simulink model "fsm_observer"  (R2025b)
settings: Solver=ode4  StartTime=0.0  StopTime=fsm_Tstop  FixedStep=fsm_h  RelTol=1e-3
values from neighbouring files (symbols this model uses):
  fsm_L1 = 0.25 * wind_p.C'    [build_fsm_observer.m]
  fsm_L2 = 0.25 * wind_p.C'    [build_fsm_observer.m]
  fsm_S = 0.05 * wind_p.C'    [build_fsm_observer.m]
  fsm_xhat0 = zeros(6, 1)    [build_fsm_observer.m]
  wind_p = wind_plant_parameters()    [build_fsm_observer.m]
settings Model: Creator=yuexi  LastModifiedBy=yuexi

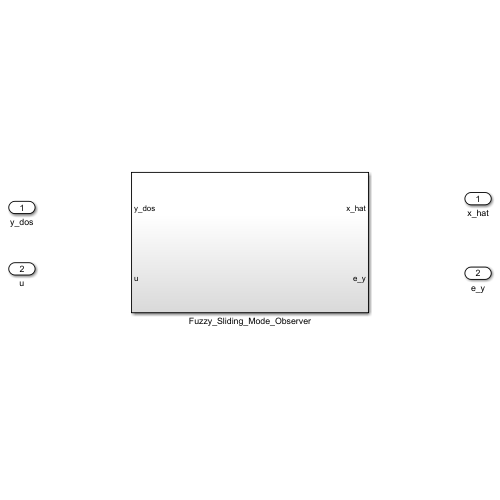
[thumbnail: Simulink's stored preview of the top-level diagram]
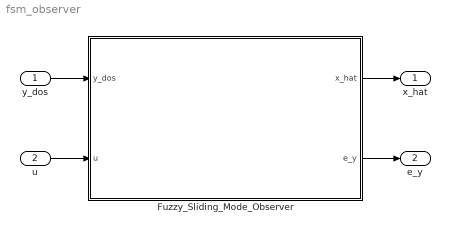
== system fsm_observer ==
  y_dos : Inport
  u : Inport  Port=2
  Fuzzy_Sliding_Mode_Observer : Subsystem
  x_hat : Outport
  e_y : Outport  Port=2
  wires:
  u/1 -> Fuzzy_Sliding_Mode_Observer/2(u)
  y_dos/1 -> Fuzzy_Sliding_Mode_Observer/1(y_dos)
  Fuzzy_Sliding_Mode_Observer/1(x_hat) -> x_hat/1
  Fuzzy_Sliding_Mode_Observer/2(e_y) -> e_y/1

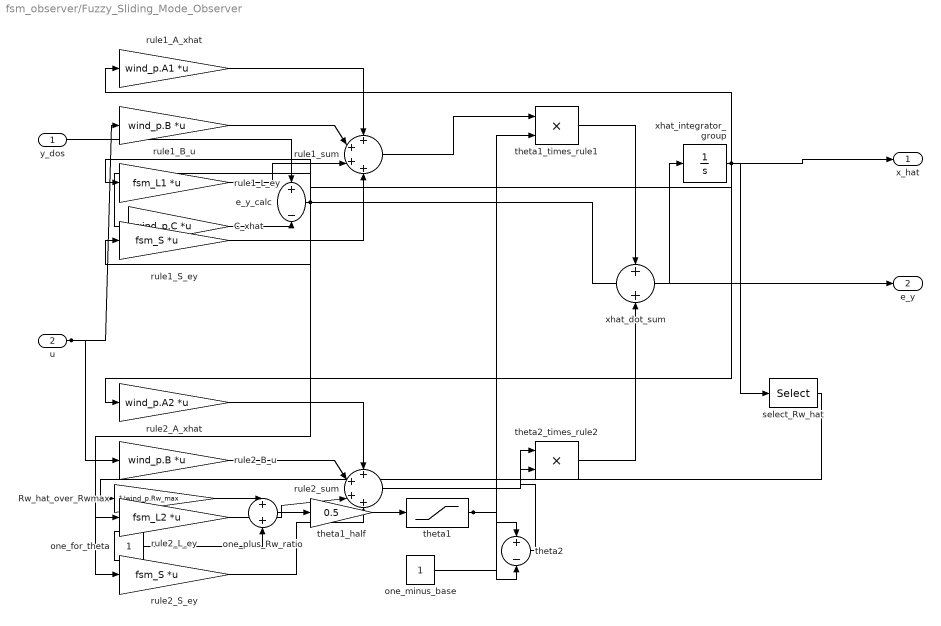
== system fsm_observer/Fuzzy_Sliding_Mode_Observer ==
  y_dos : Inport
  u : Inport  Port=2
  C_xhat : Gain  Gain=wind_p.C  Multiplication=Matrix(K*u)
  Rw_hat_over_Rwmax : Gain  Gain=1/wind_p.Rw_max
  e_y_calc : Sum  Inputs=+-
  one_for_theta : Constant
  one_minus_base : Constant
  one_plus_Rw_ratio : Sum
  rule1_A_xhat : Gain  Gain=wind_p.A1  Multiplication=Matrix(K*u)
  rule1_B_u : Gain  Gain=wind_p.B  Multiplication=Matrix(K*u)
  rule1_L_ey : Gain  Gain=fsm_L1  Multiplication=Matrix(K*u)
  rule1_S_ey : Gain  Gain=fsm_S  Multiplication=Matrix(K*u)
  rule1_sum : Sum  Inputs=++++
  rule2_A_xhat : Gain  Gain=wind_p.A2  Multiplication=Matrix(K*u)
  rule2_B_u : Gain  Gain=wind_p.B  Multiplication=Matrix(K*u)
  rule2_L_ey : Gain  Gain=fsm_L2  Multiplication=Matrix(K*u)
  rule2_S_ey : Gain  Gain=fsm_S  Multiplication=Matrix(K*u)
  rule2_sum : Sum  Inputs=++++
  select_Rw_hat : Selector  InputPortWidth=6  IndexOptions=Index vector (dialog)  Indices=6  OutputSizes=1
  theta1 : Saturate  UpperLimit=1  LowerLimit=0
  theta1_half : Gain  Gain=0.5
  theta1_times_rule1 : Product
  theta2 : Sum  Inputs=+-
  theta2_times_rule2 : Product
  xhat_dot_sum : Sum
  xhat_integrator_group : Integrator  InitialCondition=fsm_xhat0
  x_hat : Outport
  e_y : Outport  Port=2
  wires:
  xhat_integrator_group/1 -> C_xhat/1, x_hat/1, select_Rw_hat/1, rule1_A_xhat/1, rule2_A_xhat/1
  y_dos/1 -> e_y_calc/1
  C_xhat/1 -> e_y_calc/2
  e_y_calc/1 -> e_y/1, rule1_L_ey/1, rule1_S_ey/1, rule2_L_ey/1, rule2_S_ey/1
  select_Rw_hat/1 -> Rw_hat_over_Rwmax/1
  Rw_hat_over_Rwmax/1 -> one_plus_Rw_ratio/1
  one_for_theta/1 -> one_plus_Rw_ratio/2
  one_plus_Rw_ratio/1 -> theta1_half/1
  theta1_half/1 -> theta1/1
  one_minus_base/1 -> theta2/1
  theta1/1 -> theta2/2, theta1_times_rule1/2
  u/1 -> rule1_B_u/1, rule2_B_u/1
  rule1_A_xhat/1 -> rule1_sum/1
  rule1_B_u/1 -> rule1_sum/2
  rule1_L_ey/1 -> rule1_sum/3
  rule1_S_ey/1 -> rule1_sum/4
  rule2_A_xhat/1 -> rule2_sum/1
  rule2_B_u/1 -> rule2_sum/2
  rule2_L_ey/1 -> rule2_sum/3
  rule2_S_ey/1 -> rule2_sum/4
  rule1_sum/1 -> theta1_times_rule1/1
  rule2_sum/1 -> theta2_times_rule2/1
  theta2/1 -> theta2_times_rule2/2
  theta1_times_rule1/1 -> xhat_dot_sum/1
  theta2_times_rule2/1 -> xhat_dot_sum/2
  xhat_dot_sum/1 -> xhat_integrator_group/1
